simulink model "PLL_Sim_Rev1"  (R2019b)
settings: Solver=VariableStepAuto  StartTime=0.0  StopTime=10  MaxStep=100  MinStep=1e-19  RelTol=1e-2  AbsTol=1e-2
values from neighbouring files (symbols this model uses):
  C_iss = 0.1    [PLL_rev0_Plots.m]
  R = 450    [PLL_rev0_Plots.m]
  t_p = 1e-9    (= 1e-09)    [PLL_rev0_Plots.m]
  V_DD = 5    [PLL_rev0_Plots.m]
libraries: fl_lib x40, nesl_utility x21, ee_lib x15, simulink x6, simulink_extras x2, impairlib x2
settings Model: Creator=connerhannon  LastModifiedBy=connerhannon
settings SolverCC: MaxConsecutiveZCs=10000000  MaxConsecutiveMinStep=100000  ZeroCrossAlgorithm=Adaptive
settings DataIOCC: LimitDataPoints=on  MaxDataPoints=1500
settings DebuggingCC: MaxConsecutiveZCsMsg=none  MaskedZcDiagnostic=none  IgnoredZcDiagnostic=none  ArithmeticOperatorsInVariantConditions=none
settings HardwareCC: ProdBitPerLong=64  ProdHWDeviceType=Intel->x86-64 (Mac OS X)
settings ModelReferenceCC: PropagateSignalLabelsOutOfModel=off
settings SFSimCC: CustomCodeUndefinedFunction=UseInterfaceOnly
settings CodeAppCC: StateflowObjectComments=on
settings SimscapeCC: SimscapeLogType=all  SimscapeLogSimulationStatistics=on  SimscapeLogDataHistory=15000

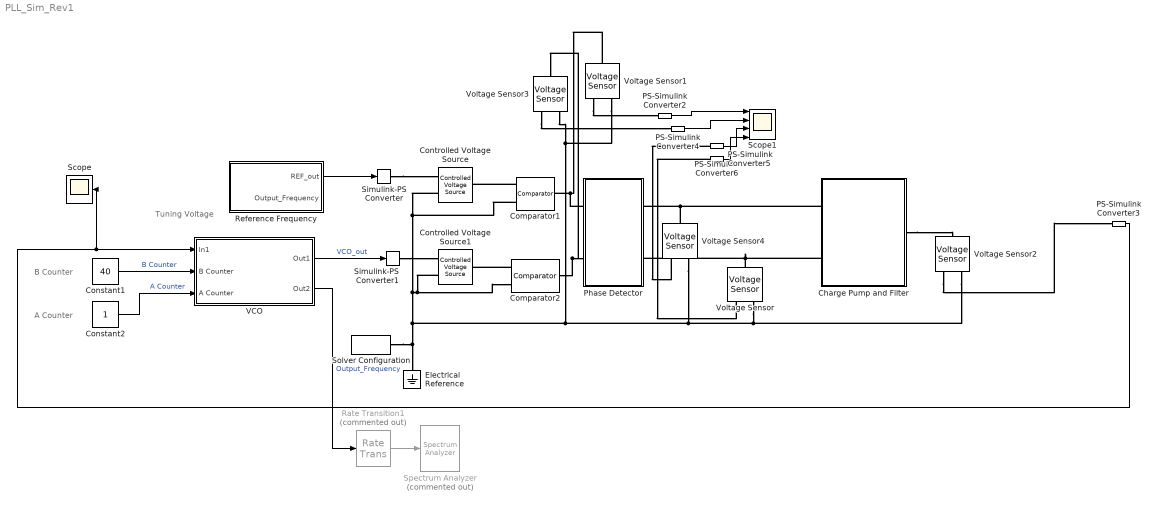
== system PLL_Sim_Rev1 ==
  note: Tuning Voltage
  note: A Counter
  note: B Counter
  Charge Pump and Filter : Subsystem  Tag=PublishSubsystem
  Comparator1 : ee_lib/Integrated Circuits/Comparator  V_OS=0 mV  V_OL=0 V  V_OH=V_DD V  C_IN=C_iss pF  R_OUT=R Ohm  Delay=t_p s
      settings: SourceProductName=Simscape Electrical  SourceProductBaseCode=PS  InternalSimscapePortConfiguration="{\"Bottom\":[],\"Left\":[{\"id\":\"p\",\"label\":\"+\",\"type\":\"foundation.electrical.electrical\"},{\"id\":\"n\",\"label\":\"-\",\"type\":\"foundation.electrical.electrical\"}],\"Right\":[{\"id\":\"J\",\"label\":\"\",\"type\":\"foundation.electrical.electrical\"}],\"Top\":[]}"
  Comparator2 : ee_lib/Integrated Circuits/Comparator  V_OS=0 mV  V_OL=0 V  V_OH=V_DD V  C_IN=C_iss pF  R_OUT=R Ohm  Delay=t_p s
      settings: SourceProductName=Simscape Electrical  SourceProductBaseCode=PS  InternalSimscapePortConfiguration="{\"Bottom\":[],\"Left\":[{\"id\":\"p\",\"label\":\"+\",\"type\":\"foundation.electrical.electrical\"},{\"id\":\"n\",\"label\":\"-\",\"type\":\"foundation.electrical.electrical\"}],\"Right\":[{\"id\":\"J\",\"label\":\"\",\"type\":\"foundation.electrical.electrical\"}],\"Top\":[]}"
  Constant1 : Constant  Value=40
  Constant2 : Constant
  Controlled Voltage Source : fl_lib/Electrical/Electrical Sources/Controlled Voltage Source
  Controlled Voltage Source1 : fl_lib/Electrical/Electrical Sources/Controlled Voltage Source
  Electrical Reference : fl_lib/Electrical/Electrical Elements/Electrical Reference
  PS-Simulink Converter{2..6} (5 alike) : nesl_utility/PS-Simulink Converter  PhysicalDomain=network_engine_domain  SubClassName=ps_output  LeftPortType=input  RightPortType=output  PseudoPeriodic=off  Frequencies=[]  Unit=inherit  AffineConversion=off
  Phase Detector : Subsystem  Tag=PublishSubsystem
  Rate Transition1 : RateTransition  Commented=on  OutPortSampleTime=1e-9
  Reference Frequency : Subsystem
  Scope : Scope
  Scope1 : Scope  NumInputPorts=4
  Simulink-PS Converter : nesl_utility/Simulink-PS Converter  PhysicalDomain=network_engine_domain  SubClassName=ps_input  LeftPortType=input  RightPortType=output  PseudoPeriodic=off  Frequencies=[]  NoiseDistribution=none  NoiseParameters=[]  Unit=1  AffineConversion=off  FilteringAndDerivatives=provide  SimscapeFilterOrder=1  InputFilterTimeConstant=0.001  UdotUserProvided=0
  Simulink-PS Converter1 : nesl_utility/Simulink-PS Converter  PhysicalDomain=network_engine_domain  SubClassName=ps_input  LeftPortType=input  RightPortType=output  PseudoPeriodic=off  Frequencies=[]  NoiseDistribution=none  NoiseParameters=[]  Unit=1  AffineConversion=off  FilteringAndDerivatives=provide  SimscapeFilterOrder=1  InputFilterTimeConstant=0.001  UdotUserProvided=0
  Solver Configuration : nesl_utility/Solver Configuration  PhysicalDomain=network_engine_domain  SubClassName=solver  LeftPortType=input  RightPortType=generic  Tones=[]  Harmonics=[]  SimulateNoise=off  Profile=off  UseLocalSampling=off  EnableSwitchedLinearOptims=on  FrequencyDomain=off  UseCCode=off  RelTol=0.001  AbsTol=1e-06  MinStep=1e-09  ToWorkspace=off  RevertToSquareIcSolve=off  NumHomotopyIterations=100  PhasorMode=off  PhasorModeNumHarmonics=1  DoDC=off  ResidualTolerance=1e-6  UseLocalSolver=off  LocalSolverChoice=NE_TRAPEZOIDAL_ADVANCER  LocalSolverSampleTime=1e-9  DoFixedCost=off  MaxNonlinIter=3  MaxModeIter=2  LinearAlgebra=auto  EquationFormulation=NE_TIME_EF  DelaysMemoryBudget=1024  AutomaticFiltering=on  FilteringTimeConstant=0.0001  PartitionStorageMethod=AS_NEEDED  PartitionMemoryBudget=1024  PartitionMethod=FAST
  Spectrum Analyzer : SpectrumAnalyzer  Commented=on
  VCO : Subsystem
  Voltage Sensor{,1..4} (5 alike) : fl_lib/Electrical/Electrical Sensors/Voltage Sensor
  wires:
  VCO/2(Out2) -> Rate Transition1/1  "Output_Frequency"
  Reference Frequency/1(REF_out) -> Simulink-PS Converter/1
  VCO/1(Out1) -> Simulink-PS Converter1/1  "VCO_out"
  Rate Transition1/1 -> Spectrum Analyzer/1
  PS-Simulink Converter2/1 -> Scope1/1
  PS-Simulink Converter4/1 -> Scope1/2
  PS-Simulink Converter6/1 -> Scope1/3
  PS-Simulink Converter5/1 -> Scope1/4
  Constant1/1 -> VCO/2(B Counter)  "B Counter"
  Constant2/1 -> VCO/3(A Counter)  "A Counter"
  PS-Simulink Converter3/1 -> Scope/1, VCO/1(In1)
  connections:
  Simulink-PS Converter1/RConn1 -- Controlled Voltage Source1/RConn1
  Simulink-PS Converter/RConn1 -- Controlled Voltage Source/RConn1
  Comparator2/LConn1 -- Controlled Voltage Source1/LConn1
  Comparator1/LConn1 -- Controlled Voltage Source/LConn1
  Phase Detector/LConn1 -- Comparator1/RConn1 -- Voltage Sensor1/LConn1
  Charge Pump and Filter/RConn1 -- Voltage Sensor2/LConn1
  Voltage Sensor2/RConn1 -- PS-Simulink Converter3/LConn1
  Charge Pump and Filter/LConn1 -- Voltage Sensor4/LConn1 -- Phase Detector/RConn1
  Charge Pump and Filter/LConn2 -- Voltage Sensor/LConn1 -- Phase Detector/RConn2
  Voltage Sensor1/RConn1 -- PS-Simulink Converter2/LConn1
  Comparator2/RConn1 -- Voltage Sensor3/LConn1 -- Phase Detector/LConn2
  Voltage Sensor3/RConn1 -- PS-Simulink Converter4/LConn1
  Voltage Sensor2/RConn2 -- Voltage Sensor/RConn2 -- Voltage Sensor4/RConn2 -- Voltage Sensor1/RConn2 -- Voltage Sensor3/RConn2 -- Comparator1/LConn2 -- Controlled Voltage Source/RConn2 -- Comparator2/LConn2 -- Controlled Voltage Source1/RConn2 -- Solver Configuration/RConn1 -- Electrical Reference/LConn1
  PS-Simulink Converter6/LConn1 -- Voltage Sensor4/RConn1
  PS-Simulink Converter5/LConn1 -- Voltage Sensor/RConn1

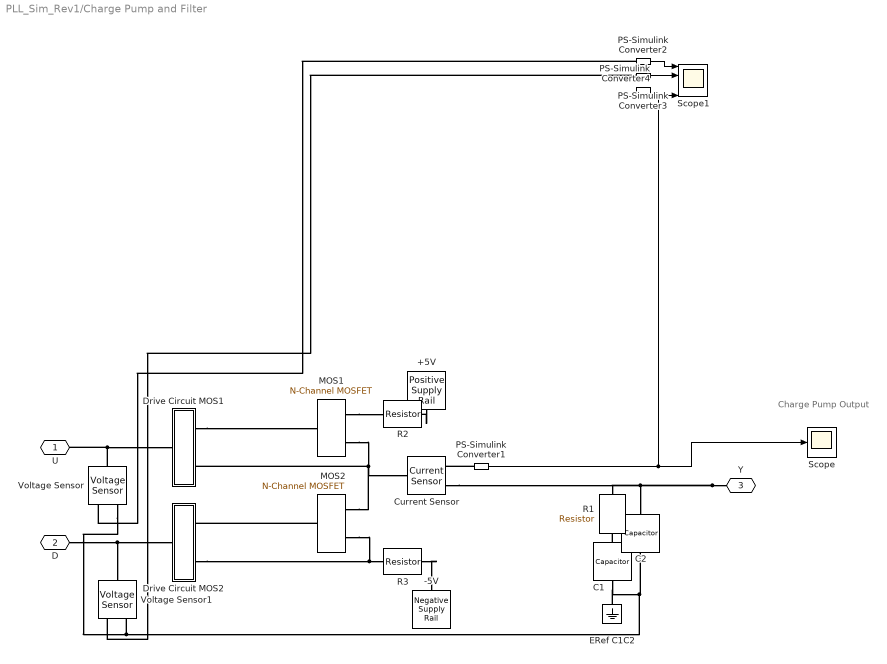
== system PLL_Sim_Rev1/Charge Pump and Filter ==
  note: Charge Pump Output
  "+5V " : ee_lib/Sources/Positive Supply Rail  v0=10 V
      settings: SourceProductName=Simscape Electrical  SourceProductBaseCode=PS  InternalSimscapePortConfiguration="{\"Bottom\":[],\"Left\":[],\"Right\":[{\"id\":\"p\",\"label\":\"\",\"type\":\"foundation.electrical.electrical\"}],\"Top\":[]}"
  -5V : ee_lib/Sources/Negative Supply Rail  v0=-10 V
      settings: SourceProductName=Simscape Electrical  SourceProductBaseCode=PS  InternalSimscapePortConfiguration="{\"Bottom\":[],\"Left\":[{\"id\":\"n\",\"label\":\"\",\"type\":\"foundation.electrical.electrical\"}],\"Right\":[],\"Top\":[]}"
  C1 : fl_lib/Electrical/Electrical Elements/Capacitor  c=82 pF  r=1e-6 Ohm  g=0 1/Ohm  i_specify=off  i_priority=High  i=0 A  i_nominal_specify=off  i_nominal_unit=A  i_nominal_value=1  v_specify=off  v_priority=High  v=0 V  v_nominal_specify=off  v_nominal_unit=V  v_nominal_value=1  vc_specify=on  vc_priority=High  vc=1 V  vc_nominal_specify=off  vc_nominal_unit=V  vc_nominal_value=1
  C2 : fl_lib/Electrical/Electrical Elements/Capacitor  c=17 pF  r=1e-6 Ohm  g=0 1/Ohm  i_specify=off  i_priority=High  i=0 A  i_nominal_specify=off  i_nominal_unit=A  i_nominal_value=1  v_specify=off  v_priority=High  v=0 V  v_nominal_specify=off  v_nominal_unit=V  v_nominal_value=1  vc_specify=on  vc_priority=High  vc=1 V  vc_nominal_specify=off  vc_nominal_unit=V  vc_nominal_value=1
  Current Sensor : fl_lib/Electrical/Electrical Sensors/Current Sensor
  Drive Circuit MOS1 : Subsystem
  Drive Circuit MOS2 : Subsystem
  ERef C1C2 : fl_lib/Electrical/Electrical Elements/Electrical Reference
  MOS1 : ee_lib/Semiconductors & Converters/N-Channel MOSFET  parameterization=1  prmDatasheet=1  prmEquCoeff=1  Beta=5 A/V^2  Rds=1000 Ohm  Id=2.5e-4 A  Vgs=5 V  Vth=1 V  lam=0 1/V  Tmeas=25 degC  RS=1 Ohm  RD=1 Ohm  C_param=1  C_GS=270 pF  C_GD=80 pF  C_DS=0 pF  C_iss=0.35 pF  C_rss=0.1 pF  C_oss=0 pF  C_GS_vec=[ 270 300 290 280 295 255 ] pF  C_GD_vec=[ 450 400 300 190 95 55 ] pF  C_DS_vec=[ 450 410 390 230 175 115 ] pF  C_iss_vec=[ 720 700 590 470 390 310 ] pF  C_rss_vec=[ 450 400 300 190 95 55 ] pF  C_oss_vec=[ 900 810 690 420 270 170 ] pF  C_Vds_vec=[ 0.1 0.3 1 3 10 30 ] V  V_GS_for_cap_data=NaN V  charge_linearity_param=1  C_OX=200 pF  V_C_OX=-0.5 V  IsDiode=0 A  Vbi=0.6 V  n=1  Cj0Diode=0 pF  TT=50e-9 s  dVth_dT=-6 mV/K  Rds_T2=0.037 Ohm  Tmeas2=125 degC  BEXDatasheet=-1.5  BEXEquCoeff=-1.5  etaisDatasheet=3  etaisEquCoeff=3  TdeviceDatasheet=25 degC  TdeviceEquCoeff=25 degC  thermal_network_parameterization=ee.enum.thermalNetworkTopology.cauer  Rth=[0, 10] K/W  Rth_Foster=[4, 6] K/W  thermal_mass_parameterization=ee.enum.thermalNetwork.timeconstant  thermal_mass=[0, 1] J/K  thermal_mass_Foster=[1.5, 3] J/K  thermal_time_constant=[0, 10] s  thermal_time_constant_Foster=[6, 18] s  thermal_mass_initial_temperatures=[25, 25] degC  betaref=18 A/V^2  Vfbref=-1.1 V  gamma=3.5 V^0.50000  phib2ref=1 V  thesatref=0.4 1/V  alpha=0  Vp=5e-2 V  thesrref=0 1/V  m=8  Tref=25 degC  Cox=1500 pF  Cgso=100 pF  Cgdo=14 pF  Rsref=2e-3 Ohm  Rdref=0.17 Ohm  Rgref=8.4 Ohm  Isref=5.2e-13 A  Cj0=480 pF  Tprm=1  etabet=1.3  Stvfb=5e-4 V/K  Stphib=-8.5e-4 V/K  etasat=1.04  etasr=0.65  etar=0.95  etais=3  Tsim=25 degC  T0=[25, 25] degC
      settings: SourceProductName=Simscape Electrical
  MOS2 : ee_lib/Semiconductors & Converters/N-Channel MOSFET  parameterization=1  prmDatasheet=1  prmEquCoeff=1  Beta=5 A/V^2  Rds=1000 Ohm  Id=2.5e-4 A  Vgs=5 V  Vth=1 V  lam=0 1/V  Tmeas=25 degC  RS=1 Ohm  RD=1 Ohm  C_param=1  C_GS=270 pF  C_GD=80 pF  C_DS=0 pF  C_iss=0.35 pF  C_rss=0.1 pF  C_oss=0 pF  C_GS_vec=[ 270 300 290 280 295 255 ] pF  C_GD_vec=[ 450 400 300 190 95 55 ] pF  C_DS_vec=[ 450 410 390 230 175 115 ] pF  C_iss_vec=[ 720 700 590 470 390 310 ] pF  C_rss_vec=[ 450 400 300 190 95 55 ] pF  C_oss_vec=[ 900 810 690 420 270 170 ] pF  C_Vds_vec=[ 0.1 0.3 1 3 10 30 ] V  V_GS_for_cap_data=NaN V  charge_linearity_param=1  C_OX=200 pF  V_C_OX=-0.5 V  IsDiode=0 A  Vbi=0.6 V  n=1  Cj0Diode=0 pF  TT=50e-9 s  dVth_dT=-6 mV/K  Rds_T2=0.037 Ohm  Tmeas2=125 degC  BEXDatasheet=-1.5  BEXEquCoeff=-1.5  etaisDatasheet=3  etaisEquCoeff=3  TdeviceDatasheet=25 degC  TdeviceEquCoeff=25 degC  thermal_network_parameterization=ee.enum.thermalNetworkTopology.cauer  Rth=[0, 10] K/W  Rth_Foster=[4, 6] K/W  thermal_mass_parameterization=ee.enum.thermalNetwork.timeconstant  thermal_mass=[0, 1] J/K  thermal_mass_Foster=[1.5, 3] J/K  thermal_time_constant=[0, 10] s  thermal_time_constant_Foster=[6, 18] s  thermal_mass_initial_temperatures=[25, 25] degC  betaref=18 A/V^2  Vfbref=-1.1 V  gamma=3.5 V^0.50000  phib2ref=1 V  thesatref=0.4 1/V  alpha=0  Vp=5e-2 V  thesrref=0 1/V  m=8  Tref=25 degC  Cox=1500 pF  Cgso=100 pF  Cgdo=14 pF  Rsref=2e-3 Ohm  Rdref=0.17 Ohm  Rgref=8.4 Ohm  Isref=5.2e-13 A  Cj0=480 pF  Tprm=1  etabet=1.3  Stvfb=5e-4 V/K  Stphib=-8.5e-4 V/K  etasat=1.04  etasr=0.65  etar=0.95  etais=3  Tsim=25 degC  T0=[25, 25] degC
      settings: SourceProductName=Simscape Electrical
  PS-Simulink Converter{1..4} (4 alike) : nesl_utility/PS-Simulink Converter  PhysicalDomain=network_engine_domain  SubClassName=ps_output  LeftPortType=input  RightPortType=output  PseudoPeriodic=off  Frequencies=[]  Unit=inherit  AffineConversion=off
  R1 : ee_lib/Passive/Resistor  R=23 kOhm  R_tol=5  enable_R_tol=0  tol_distribution=1  nSigma=4  enable_operating_limits=0  operating_limit_action=2  max_working_voltage=100 V  power_rating=1 W  enable_faults=0  fault_action=1  R_faulted=Inf Ohm  enable_temporal_fault=0  t_fault=1 s  enable_behavioral_fault=0  max_permissible_current=1 A  t_fail_on_current=1 s  noise_mode=0  sample_time=0.001 s  repeatability=1  auto_seed=66516699  user_seed=0  Tdevice=25 degC  alpha=3.93e-3 1/K  Tmeas=25 degC  thermal_mass=100 J/K  power_derating_T1=70 degC  power_derating_T2=155 degC  operating_temperature_range_vec=[-50, 150] degC  temperature_specify=off  temperature_priority=High  temperature=298.15 K  temperature_nominal_specify=off  temperature_nominal_unit=K  temperature_nominal_value=1
      settings: SourceProductName=Simscape Electrical
  R2 : ee_lib/Passive/Resistor  R=40 kOhm  R_tol=5  enable_R_tol=0  tol_distribution=1  nSigma=4  enable_operating_limits=0  operating_limit_action=2  max_working_voltage=100 V  power_rating=1 W  enable_faults=0  fault_action=1  R_faulted=Inf Ohm  enable_temporal_fault=0  t_fault=1 s  enable_behavioral_fault=0  max_permissible_current=1 A  t_fail_on_current=1 s  noise_mode=0  sample_time=0.001 s  repeatability=1  auto_seed=4226521513  user_seed=0  Tdevice=25 degC  alpha=3.93e-3 1/K  Tmeas=25 degC  thermal_mass=100 J/K  power_derating_T1=70 degC  power_derating_T2=155 degC  operating_temperature_range_vec=[-50, 150] degC  temperature_specify=off  temperature_priority=High  temperature=298.15 K  temperature_nominal_specify=off  temperature_nominal_unit=K  temperature_nominal_value=1
      settings: SourceProductName=Simscape Electrical
  R3 : ee_lib/Passive/Resistor  R=40 kOhm  R_tol=5  enable_R_tol=0  tol_distribution=1  nSigma=4  enable_operating_limits=0  operating_limit_action=2  max_working_voltage=100 V  power_rating=1 W  enable_faults=0  fault_action=1  R_faulted=Inf Ohm  enable_temporal_fault=0  t_fault=1 s  enable_behavioral_fault=0  max_permissible_current=1 A  t_fail_on_current=1 s  noise_mode=0  sample_time=0.001 s  repeatability=1  auto_seed=717982854  user_seed=0  Tdevice=25 degC  alpha=3.93e-3 1/K  Tmeas=25 degC  thermal_mass=100 J/K  power_derating_T1=70 degC  power_derating_T2=155 degC  operating_temperature_range_vec=[-50, 150] degC  temperature_specify=off  temperature_priority=High  temperature=298.15 K  temperature_nominal_specify=off  temperature_nominal_unit=K  temperature_nominal_value=1
      settings: SourceProductName=Simscape Electrical
  Scope : Scope
  Scope1 : Scope  NumInputPorts=4
  Voltage Sensor : fl_lib/Electrical/Electrical Sensors/Voltage Sensor
  Voltage Sensor1 : fl_lib/Electrical/Electrical Sensors/Voltage Sensor
  U : PMIOPort  Side=Left
  D : PMIOPort  Port=2  Side=Left
  Y : PMIOPort  Port=3  Side=Right
  wires:
  PS-Simulink Converter1/1 -> Scope1/4, Scope/1
  PS-Simulink Converter2/1 -> Scope1/1
  PS-Simulink Converter3/1 -> Scope1/2
  connections:
  C1/LConn1 -- R1/RConn1
  MOS2/RConn2 -- Drive Circuit MOS2/RConn2 -- R3/LConn1
  "+5V "/RConn1 -- R2/LConn1
  MOS1/RConn1 -- R2/RConn1
  R3/RConn1 -- -5V/LConn1
  MOS1/RConn2 -- MOS2/RConn1 -- Current Sensor/LConn1 -- Drive Circuit MOS1/RConn2
  PS-Simulink Converter1/LConn1 -- Current Sensor/RConn1
  Voltage Sensor/RConn2 -- C2/RConn1 -- C1/RConn1 -- ERef C1C2/LConn1 -- Voltage Sensor1/RConn2
  MOS2/LConn1 -- Drive Circuit MOS2/RConn1
  Drive Circuit MOS1/RConn1 -- MOS1/LConn1
  PS-Simulink Converter2/LConn1 -- Voltage Sensor/RConn1
  PS-Simulink Converter3/LConn1 -- Voltage Sensor1/RConn1
  Voltage Sensor/LConn1 -- Drive Circuit MOS1/LConn1 -- U/RConn1
  D/RConn1 -- Voltage Sensor1/LConn1 -- Drive Circuit MOS2/LConn1
  Y/RConn1 -- Current Sensor/RConn2 -- R1/LConn1 -- C2/LConn1

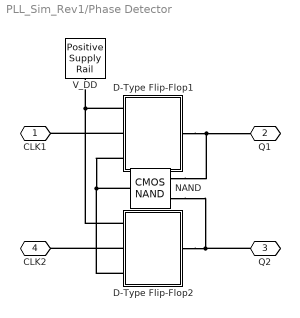
== system PLL_Sim_Rev1/Phase Detector ==
  D-Type Flip-Flop1 : Subsystem  mask(D-Type Flip-Flop){C_iss=C_iss, t_p=t_p, V_DD=V_DD, R=R}
      mask prompts: C_iss "Gate input capacitance (pF)"; t_p "Gate propagation delay (s)"; V_DD "Supply voltage (V)"; R "Gate effective output resistance (ohms)"
      mask help: Behavioral model of a D-type flip-flop built from Simscape(TM) Electrical(TM) library components.
  D-Type Flip-Flop2 : Subsystem  mask(D-Type Flip-Flop){C_iss=C_iss, t_p=t_p, V_DD=V_DD, R=R}
      mask prompts: C_iss "Gate input capacitance (pF)"; t_p "Gate propagation delay (s)"; V_DD "Supply voltage (V)"; R "Gate effective output resistance (ohms)"
      mask help: Behavioral model of a D-type flip-flop built from Simscape(TM) Electrical(TM) library components.
  NAND : ee_lib/Integrated Circuits/Logic/CMOS NAND  V_IL=0.4*V_DD V  V_IH=0.6*V_DD V  C_IN=C_iss pF  output_type=1  V_OL=0 V  V_OH=V_DD V  V_CC=5 V  V_meas=5 V  R_OUT=R Ohm  R_OH=[ 25 250 ] Ohm  I_OH=63 mA  R_OL=[ 30 800 ] Ohm  I_OL=-45 mA  Delay=t_p s  Ron=5 Ohm  Vf=0.6 V  output_state=1
      settings: SourceProductName=Simscape Electrical  SourceProductBaseCode=PS  InternalSimscapePortConfiguration="{\"Bottom\":[],\"Left\":[{\"id\":\"A\",\"label\":\"\",\"type\":\"foundation.electrical.electrical\"},{\"id\":\"B\",\"label\":\"\",\"type\":\"foundation.electrical.electrical\"}],\"Right\":[{\"id\":\"J\",\"label\":\"\",\"type\":\"foundation.electrical.electrical\"}],\"Top\":[]}"
  V_DD : ee_lib/Sources/Positive Supply Rail  v0=V_DD V
      settings: SourceProductName=Simscape Electrical  SourceProductBaseCode=PS  InternalSimscapePortConfiguration="{\"Bottom\":[],\"Left\":[],\"Right\":[{\"id\":\"p\",\"label\":\"\",\"type\":\"foundation.electrical.electrical\"}],\"Top\":[]}"
  CLK1 : PMIOPort  Side=Left
  Q1 : PMIOPort  Port=2  Side=Right
  Q2 : PMIOPort  Port=3  Side=Right
  CLK2 : PMIOPort  Port=4  Side=Left
  connections:
  D-Type Flip-Flop1/LConn1 -- D-Type Flip-Flop2/LConn1 -- V_DD/RConn1
  D-Type Flip-Flop1/LConn3 -- D-Type Flip-Flop2/LConn3 -- NAND/RConn1
  NAND/LConn2 -- D-Type Flip-Flop1/RConn1 -- Q1/RConn1
  NAND/LConn1 -- D-Type Flip-Flop2/RConn1 -- Q2/RConn1
  D-Type Flip-Flop2/LConn2 -- CLK2/RConn1
  D-Type Flip-Flop1/LConn2 -- CLK1/RConn1

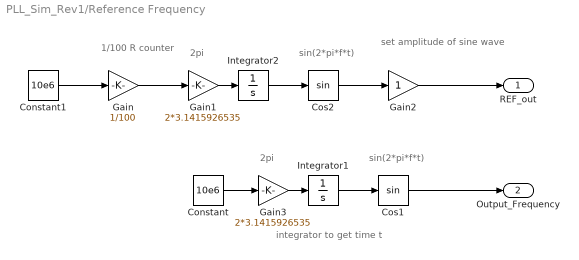
== system PLL_Sim_Rev1/Reference Frequency ==
  note: set amplitude of sine wave
  note: 1/100
      | R counter
  note: integrator to get time t
  note: sin(2*pi*f*t)
  note: 2pi
  note: sin(2*pi*f*t)
  note: 2pi
  Constant : Constant  Value=10e6
  Constant1 : Constant  Value=10e6
  Cos1 : Trigonometry  OutputSignalType=real
  Cos2 : Trigonometry  OutputSignalType=real
  Gain : Gain  Gain=1/100
  Gain1 : Gain  Gain=2*3.1415926535
  Gain2 : Gain
  Gain3 : Gain  Gain=2*3.1415926535
  Integrator1 : Integrator
  Integrator2 : Integrator
  REF_out : Outport
  "Output_Frequency " : Outport  Port=2
  wires:
  Cos1/1 -> "Output_Frequency "/1
  Gain3/1 -> Integrator1/1
  Integrator1/1 -> Cos1/1
  Constant/1 -> Gain3/1
  Constant1/1 -> Gain/1
  Gain1/1 -> Integrator2/1
  Integrator2/1 -> Cos2/1
  Gain/1 -> Gain1/1
  Cos2/1 -> Gain2/1
  Gain2/1 -> REF_out/1

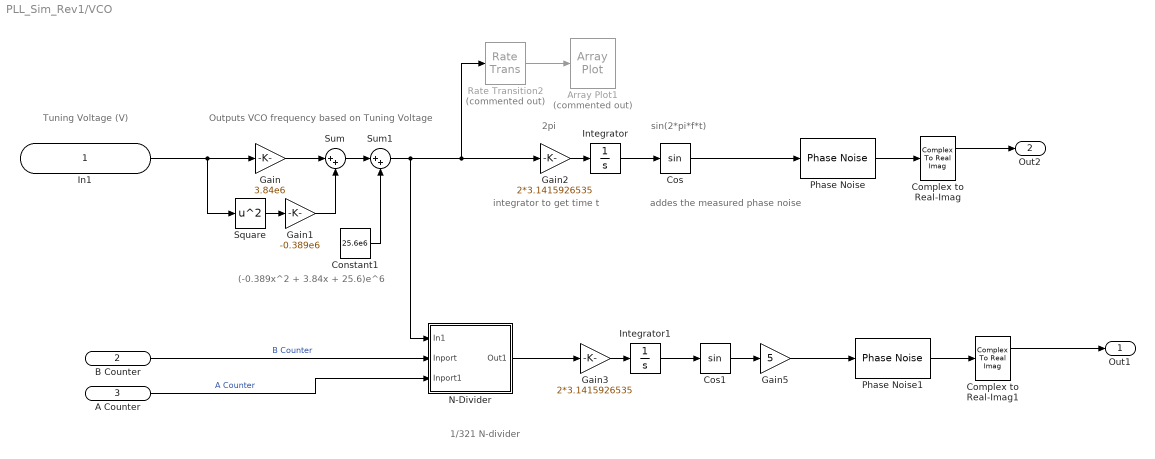
== system PLL_Sim_Rev1/VCO ==
  note: 1/321
      | N-divider
  note: Tuning Voltage
      | (V)
  note: 2pi
  note: sin(2*pi*f*t)
  note: integrator to get time t
  note: (-0.389x^2 + 3.84x + 25.6)e^6
  note: addes the measured phase noise
  note: Outputs VCO frequency based on Tuning Voltage
  In1 : Inport
  B Counter : Inport  Port=2
  A Counter : Inport  Port=3
  Array Plot1 : ArrayPlot  Commented=on
  Complex to Real-Imag : ComplexToRealImag
  Complex to Real-Imag1 : ComplexToRealImag
  Constant1 : Constant  Value=25.6e6
  Cos : Trigonometry  OutputSignalType=complex
  Cos1 : Trigonometry  OutputSignalType=complex
  Gain : Gain  Gain=3.84e6
  Gain1 : Gain  Gain=-0.389e6
  Gain2 : Gain  Gain=2*3.1415926535
  Gain3 : Gain  Gain=2*3.1415926535
  Gain5 : Gain  Gain=5
  Integrator : Integrator
  Integrator1 : Integrator
  N-Divider : Subsystem
  Phase Noise : impairlib/Phase Noise  Level=[ -36, -73, -83, -90, -112 ]  FrequencyOffset=[ 100, 400, 1000, 5000, 250000]  SampleRate=550000  RandomStream=mt19937ar with seed  Seed=1e6  SimulateUsing=Interpreted execution
      settings: SourceProductName=SerDes Toolbox  SourceProductBaseCode=SX
  Phase Noise1 : impairlib/Phase Noise  Level=[ -36, -73, -83, -90, -112 ]  FrequencyOffset=[ 100, 400, 1000, 5000, 250000]  SampleRate=550000  RandomStream=mt19937ar with seed  Seed=1e6  SimulateUsing=Interpreted execution
      settings: SourceProductName=SerDes Toolbox  SourceProductBaseCode=SX
  Rate Transition2 : RateTransition  Commented=on  OutPortSampleTime=1/1000000000
  Square : Math  Operator=square  SignedPower=off  SaturateOnIntegerOverflow=on
  Sum : Sum  Inputs=|++
  Sum1 : Sum  Inputs=|++
  Out1 : Outport
  Out2 : Outport  Port=2
  wires:
  Gain1/1 -> Sum/2
  Gain/1 -> Sum/1
  Square/1 -> Gain1/1
  Integrator/1 -> Cos/1
  Constant1/1 -> Sum1/2
  Phase Noise/1 -> Complex to Real-Imag/1
  Sum/1 -> Sum1/1
  Cos/1 -> Phase Noise/1
  In1/1 -> Square/1, Gain/1
  Gain2/1 -> Integrator/1
  Gain3/1 -> Integrator1/1
  Phase Noise1/1 -> Complex to Real-Imag1/1
  Cos1/1 -> Gain5/1
  Integrator1/1 -> Cos1/1
  Complex to Real-Imag1/1 -> Out1/1
  Complex to Real-Imag/1 -> Out2/1
  Gain5/1 -> Phase Noise1/1
  Sum1/1 -> N-Divider/1(In1), Rate Transition2/1, Gain2/1
  B Counter/1 -> N-Divider/2(Inport)  "B Counter"
  A Counter/1 -> N-Divider/3(Inport1)  "A Counter"
  N-Divider/1(Out1) -> Gain3/1
  Rate Transition2/1 -> Array Plot1/1

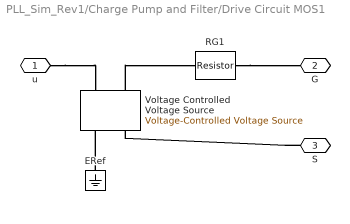
== system PLL_Sim_Rev1/Charge Pump and Filter/Drive Circuit MOS1 ==
  ERef : fl_lib/Electrical/Electrical Elements/Electrical Reference
  RG1 : ee_lib/Passive/Resistor  R=40 kOhm  R_tol=5  enable_R_tol=0  tol_distribution=1  nSigma=4  enable_operating_limits=0  operating_limit_action=2  max_working_voltage=100 V  power_rating=1 W  enable_faults=0  fault_action=1  R_faulted=Inf Ohm  enable_temporal_fault=0  t_fault=1 s  enable_behavioral_fault=0  max_permissible_current=1 A  t_fail_on_current=1 s  noise_mode=0  sample_time=0.001 s  repeatability=1  auto_seed=1254062075  user_seed=0  Tdevice=25 degC  alpha=3.93e-3 1/K  Tmeas=25 degC  thermal_mass=100 J/K  power_derating_T1=70 degC  power_derating_T2=155 degC  operating_temperature_range_vec=[-50, 150] degC  temperature_specify=off  temperature_priority=High  temperature=298.15 K  temperature_nominal_specify=off  temperature_nominal_unit=K  temperature_nominal_value=1
      settings: SourceProductName=Simscape Electrical
  Voltage Controlled Voltage Source : fl_lib/Electrical/Electrical Sources/Voltage-Controlled Voltage Source  K=1  v1_specify=off  v1_priority=High  v1=0 V  v1_nominal_specify=off  v1_nominal_unit=V  v1_nominal_value=1  v2_specify=off  v2_priority=High  v2=0 V  v2_nominal_specify=off  v2_nominal_unit=V  v2_nominal_value=1
      settings: SourceProductName=Simscape  SourceProductBaseCode=SS  InternalSimscapePortConfiguration="{\"Bottom\":[],\"Left\":[{\"id\":\"p1\",\"label\":\"+\",\"type\":\"foundation.electrical.electrical\"},{\"id\":\"p2\",\"label\":\"+\",\"type\":\"foundation.electrical.electrical\"}],\"Right\":[{\"id\":\"n1\",\"label\":\"-\",\"type\":\"foundation.electrical.electrical\"},{\"id\":\"n2\",\"label\":\"-\",\"type\":\"foundation.electrical.electrical\"}],\"Top\":[]}"
  u : PMIOPort  Side=Left
  G : PMIOPort  Port=2  Side=Right
  S : PMIOPort  Port=3  Side=Right
  connections:
  u/RConn1 -- Voltage Controlled Voltage Source/LConn1
  S/RConn1 -- Voltage Controlled Voltage Source/RConn2
  RG1/RConn1 -- G/RConn1
  Voltage Controlled Voltage Source/LConn2 -- RG1/LConn1
  ERef/LConn1 -- Voltage Controlled Voltage Source/RConn1

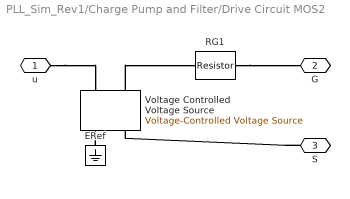
== system PLL_Sim_Rev1/Charge Pump and Filter/Drive Circuit MOS2 ==
  ERef : fl_lib/Electrical/Electrical Elements/Electrical Reference
  RG1 : ee_lib/Passive/Resistor  R=40 kOhm  R_tol=5  enable_R_tol=0  tol_distribution=1  nSigma=4  enable_operating_limits=0  operating_limit_action=2  max_working_voltage=100 V  power_rating=1 W  enable_faults=0  fault_action=1  R_faulted=Inf Ohm  enable_temporal_fault=0  t_fault=1 s  enable_behavioral_fault=0  max_permissible_current=1 A  t_fail_on_current=1 s  noise_mode=0  sample_time=0.001 s  repeatability=1  auto_seed=1853927660  user_seed=0  Tdevice=25 degC  alpha=3.93e-3 1/K  Tmeas=25 degC  thermal_mass=100 J/K  power_derating_T1=70 degC  power_derating_T2=155 degC  operating_temperature_range_vec=[-50, 150] degC  temperature_specify=off  temperature_priority=High  temperature=298.15 K  temperature_nominal_specify=off  temperature_nominal_unit=K  temperature_nominal_value=1
      settings: SourceProductName=Simscape Electrical
  Voltage Controlled Voltage Source : fl_lib/Electrical/Electrical Sources/Voltage-Controlled Voltage Source  K=1  v1_specify=off  v1_priority=High  v1=0 V  v1_nominal_specify=off  v1_nominal_unit=V  v1_nominal_value=1  v2_specify=off  v2_priority=High  v2=0 V  v2_nominal_specify=off  v2_nominal_unit=V  v2_nominal_value=1
      settings: SourceProductName=Simscape  SourceProductBaseCode=SS  InternalSimscapePortConfiguration="{\"Bottom\":[],\"Left\":[{\"id\":\"p1\",\"label\":\"+\",\"type\":\"foundation.electrical.electrical\"},{\"id\":\"p2\",\"label\":\"+\",\"type\":\"foundation.electrical.electrical\"}],\"Right\":[{\"id\":\"n1\",\"label\":\"-\",\"type\":\"foundation.electrical.electrical\"},{\"id\":\"n2\",\"label\":\"-\",\"type\":\"foundation.electrical.electrical\"}],\"Top\":[]}"
  u : PMIOPort  Side=Left
  G : PMIOPort  Port=2  Side=Right
  S : PMIOPort  Port=3  Side=Right
  connections:
  ERef/LConn1 -- Voltage Controlled Voltage Source/RConn1
  Voltage Controlled Voltage Source/LConn2 -- RG1/LConn1
  RG1/RConn1 -- G/RConn1
  S/RConn1 -- Voltage Controlled Voltage Source/RConn2
  u/RConn1 -- Voltage Controlled Voltage Source/LConn1

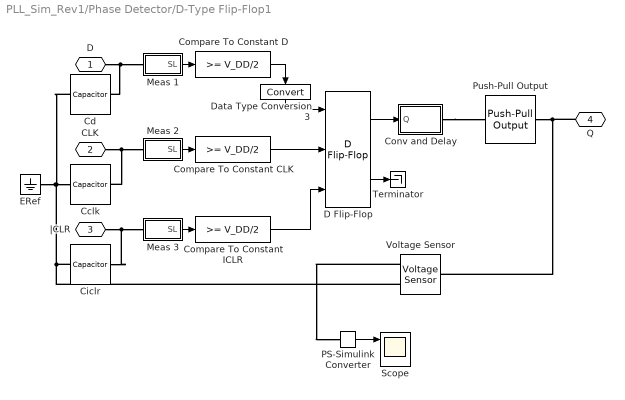
== system PLL_Sim_Rev1/Phase Detector/D-Type Flip-Flop1 ==
  Cclk : fl_lib/Electrical/Electrical Elements/Capacitor  c=C_iss pF  r=1e-06 Ohm  g=0 1/Ohm  i_specify=off  i_priority=High  i=0 A  i_nominal_specify=off  i_nominal_unit=A  i_nominal_value=1  v_specify=off  v_priority=High  v=0 V  v_nominal_specify=off  v_nominal_unit=V  v_nominal_value=1  vc_specify=on  vc_priority=High  vc=0 V  vc_nominal_specify=off  vc_nominal_unit=V  vc_nominal_value=1
  Cd : fl_lib/Electrical/Electrical Elements/Capacitor  c=C_iss pF  r=1e-06 Ohm  g=0 1/Ohm  i_specify=off  i_priority=High  i=0 A  i_nominal_specify=off  i_nominal_unit=A  i_nominal_value=1  v_specify=off  v_priority=High  v=0 V  v_nominal_specify=off  v_nominal_unit=V  v_nominal_value=1  vc_specify=on  vc_priority=High  vc=0 V  vc_nominal_specify=off  vc_nominal_unit=V  vc_nominal_value=1
  Ciclr : fl_lib/Electrical/Electrical Elements/Capacitor  c=C_iss pF  r=1e-06 Ohm  g=0 1/Ohm  i_specify=off  i_priority=High  i=0 A  i_nominal_specify=off  i_nominal_unit=A  i_nominal_value=1  v_specify=off  v_priority=High  v=0 V  v_nominal_specify=off  v_nominal_unit=V  v_nominal_value=1  vc_specify=on  vc_priority=High  vc=0 V  vc_nominal_specify=off  vc_nominal_unit=V  vc_nominal_value=1
  Compare To Constant CLK : simulink/Logic and Bit Operations/Compare To Constant  relop=>=  const=V_DD/2  OutDataTypeStr=boolean
  Compare To Constant D : simulink/Logic and Bit Operations/Compare To Constant  relop=>=  const=V_DD/2  OutDataTypeStr=boolean
  Compare To Constant ICLR : simulink/Logic and Bit Operations/Compare To Constant  relop=>=  const=V_DD/2  OutDataTypeStr=boolean
  Conv and Delay : Subsystem
  D Flip-Flop : simulink_extras/Flip Flops/D Flip-Flop
      settings: SourceProductName=Simulink
  Data Type Conversion3 : DataTypeConversion
  ERef : fl_lib/Electrical/Electrical Elements/Electrical Reference
  Meas 1 : Subsystem
  Meas 2 : Subsystem
  Meas 3 : Subsystem
  PS-Simulink Converter : nesl_utility/PS-Simulink Converter  PhysicalDomain=network_engine_domain  SubClassName=ps_output  LeftPortType=input  RightPortType=output  PseudoPeriodic=off  Frequencies=[]  Unit=inherit  AffineConversion=off
  Push-Pull Output : ee_lib/Integrated Circuits/Push-Pull Output  k=-V_DD V  c=-1  output_type=1  V_neg=0 V  V_pos=V_DD V  V_meas=[ 0 5 ] V  R_OUT=R Ohm  R_OH=[ 25 250 ] Ohm  I_OH=63 mA  R_OL=[ 30 800 ] Ohm  I_OL=-45 mA  Delay=0 s  Ron=5 Ohm  Vf=0.6 V  V0=0 V  X0=0
      settings: SourceProductName=Simscape Electrical  SourceProductBaseCode=PS  InternalSimscapePortConfiguration="{\"Bottom\":[],\"Left\":[{\"id\":\"X\",\"label\":\"X\",\"type\":\"input\"}],\"Right\":[{\"id\":\"J\",\"label\":\"\",\"type\":\"foundation.electrical.electrical\"}],\"Top\":[]}"
  Scope : Scope  NumInputPorts=3
  Terminator : Terminator
  Voltage Sensor : fl_lib/Electrical/Electrical Sensors/Voltage Sensor
  D : PMIOPort  Side=Left
  CLK : PMIOPort  Port=2  Side=Left
  |CLR : PMIOPort  Port=3  Side=Left
  Q : PMIOPort  Port=4  Side=Right
  wires:
  Data Type Conversion3/1 -> D Flip-Flop/1
  Compare To Constant ICLR/1 -> D Flip-Flop/3
  Compare To Constant CLK/1 -> D Flip-Flop/2
  D Flip-Flop/2 -> Terminator/1
  Compare To Constant D/1 -> Data Type Conversion3/1
  Meas 3/1(SL) -> Compare To Constant ICLR/1
  Meas 2/1(SL) -> Compare To Constant CLK/1
  Meas 1/1(SL) -> Compare To Constant D/1
  D Flip-Flop/1 -> Conv and Delay/1(Q)
  PS-Simulink Converter/1 -> Scope/1
  connections:
  |CLR/RConn1 -- Ciclr/LConn1 -- Meas 3/LConn1
  Voltage Sensor/LConn1 -- Q/RConn1 -- Push-Pull Output/RConn1
  CLK/RConn1 -- Meas 2/LConn1 -- Cclk/LConn1
  D/RConn1 -- Cd/LConn1 -- Meas 1/LConn1
  ERef/LConn1 -- Voltage Sensor/RConn2 -- Ciclr/RConn1 -- Cd/RConn1 -- Cclk/RConn1
  Conv and Delay/RConn1 -- Push-Pull Output/LConn1
  Voltage Sensor/RConn1 -- PS-Simulink Converter/LConn1

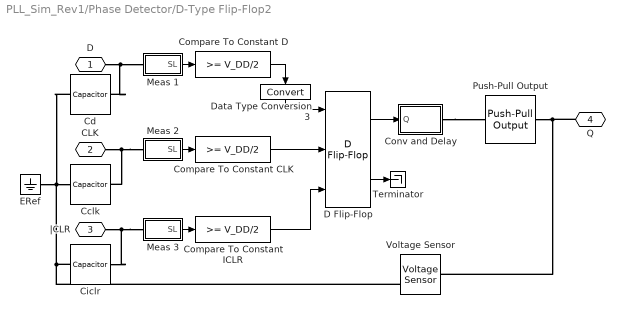
== system PLL_Sim_Rev1/Phase Detector/D-Type Flip-Flop2 ==
  Cclk : fl_lib/Electrical/Electrical Elements/Capacitor  c=C_iss pF  r=1e-06 Ohm  g=0 1/Ohm  i_specify=off  i_priority=High  i=0 A  i_nominal_specify=off  i_nominal_unit=A  i_nominal_value=1  v_specify=off  v_priority=High  v=0 V  v_nominal_specify=off  v_nominal_unit=V  v_nominal_value=1  vc_specify=on  vc_priority=High  vc=0 V  vc_nominal_specify=off  vc_nominal_unit=V  vc_nominal_value=1
  Cd : fl_lib/Electrical/Electrical Elements/Capacitor  c=C_iss pF  r=1e-06 Ohm  g=0 1/Ohm  i_specify=off  i_priority=High  i=0 A  i_nominal_specify=off  i_nominal_unit=A  i_nominal_value=1  v_specify=off  v_priority=High  v=0 V  v_nominal_specify=off  v_nominal_unit=V  v_nominal_value=1  vc_specify=on  vc_priority=High  vc=0 V  vc_nominal_specify=off  vc_nominal_unit=V  vc_nominal_value=1
  Ciclr : fl_lib/Electrical/Electrical Elements/Capacitor  c=C_iss pF  r=1e-06 Ohm  g=0 1/Ohm  i_specify=off  i_priority=High  i=0 A  i_nominal_specify=off  i_nominal_unit=A  i_nominal_value=1  v_specify=off  v_priority=High  v=0 V  v_nominal_specify=off  v_nominal_unit=V  v_nominal_value=1  vc_specify=on  vc_priority=High  vc=0 V  vc_nominal_specify=off  vc_nominal_unit=V  vc_nominal_value=1
  Compare To Constant CLK : simulink/Logic and Bit Operations/Compare To Constant  relop=>=  const=V_DD/2  OutDataTypeStr=boolean
  Compare To Constant D : simulink/Logic and Bit Operations/Compare To Constant  relop=>=  const=V_DD/2  OutDataTypeStr=boolean
  Compare To Constant ICLR : simulink/Logic and Bit Operations/Compare To Constant  relop=>=  const=V_DD/2  OutDataTypeStr=boolean
  Conv and Delay : Subsystem
  D Flip-Flop : simulink_extras/Flip Flops/D Flip-Flop
      settings: SourceProductName=Simulink
  Data Type Conversion3 : DataTypeConversion
  ERef : fl_lib/Electrical/Electrical Elements/Electrical Reference
  Meas 1 : Subsystem
  Meas 2 : Subsystem
  Meas 3 : Subsystem
  Push-Pull Output : ee_lib/Integrated Circuits/Push-Pull Output  k=-V_DD V  c=-1  output_type=1  V_neg=0 V  V_pos=V_DD V  V_meas=[ 0 5 ] V  R_OUT=R Ohm  R_OH=[ 25 250 ] Ohm  I_OH=63 mA  R_OL=[ 30 800 ] Ohm  I_OL=-45 mA  Delay=0 s  Ron=5 Ohm  Vf=0.6 V  V0=0 V  X0=0
      settings: SourceProductName=Simscape Electrical  SourceProductBaseCode=PS  InternalSimscapePortConfiguration="{\"Bottom\":[],\"Left\":[{\"id\":\"X\",\"label\":\"X\",\"type\":\"input\"}],\"Right\":[{\"id\":\"J\",\"label\":\"\",\"type\":\"foundation.electrical.electrical\"}],\"Top\":[]}"
  Terminator : Terminator
  Voltage Sensor : fl_lib/Electrical/Electrical Sensors/Voltage Sensor
  D : PMIOPort  Side=Left
  CLK : PMIOPort  Port=2  Side=Left
  |CLR : PMIOPort  Port=3  Side=Left
  Q : PMIOPort  Port=4  Side=Right
  wires:
  D Flip-Flop/1 -> Conv and Delay/1(Q)
  Meas 1/1(SL) -> Compare To Constant D/1
  Meas 2/1(SL) -> Compare To Constant CLK/1
  Meas 3/1(SL) -> Compare To Constant ICLR/1
  Compare To Constant D/1 -> Data Type Conversion3/1
  D Flip-Flop/2 -> Terminator/1
  Compare To Constant CLK/1 -> D Flip-Flop/2
  Compare To Constant ICLR/1 -> D Flip-Flop/3
  Data Type Conversion3/1 -> D Flip-Flop/1
  connections:
  Conv and Delay/RConn1 -- Push-Pull Output/LConn1
  Ciclr/RConn1 -- Voltage Sensor/RConn2 -- Cclk/RConn1 -- ERef/LConn1 -- Cd/RConn1
  Cd/LConn1 -- Meas 1/LConn1 -- D/RConn1
  Meas 2/LConn1 -- Cclk/LConn1 -- CLK/RConn1
  Push-Pull Output/RConn1 -- Q/RConn1 -- Voltage Sensor/LConn1
  Meas 3/LConn1 -- |CLR/RConn1 -- Ciclr/LConn1

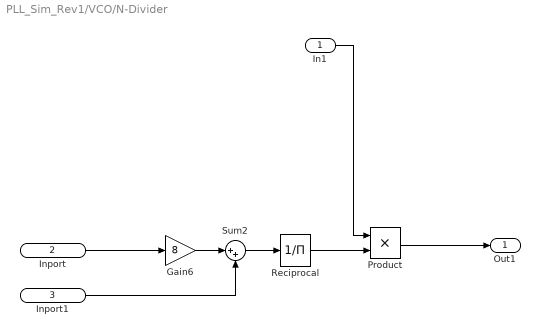
== system PLL_Sim_Rev1/VCO/N-Divider ==
  In1 : Inport
  Inport : Inport  Port=2
  Inport1 : Inport  Port=3
  Gain6 : Gain  Gain=8
  Product : Product
  Reciprocal : Product  Inputs=/
  Sum2 : Sum  Inputs=|++
  Out1 : Outport
  wires:
  Product/1 -> Out1/1
  Inport/1 -> Gain6/1
  Sum2/1 -> Reciprocal/1
  Gain6/1 -> Sum2/1
  Reciprocal/1 -> Product/2
  In1/1 -> Product/1
  Inport1/1 -> Sum2/2

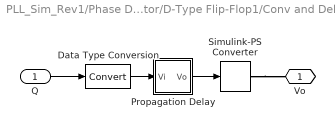
== system PLL_Sim_Rev1/Phase Detector/D-Type Flip-Flop1/Conv and Delay ==
  Q : Inport
  Data Type Conversion : DataTypeConversion
  Propagation Delay : Subsystem
  Simulink-PS Converter : nesl_utility/Simulink-PS Converter  PhysicalDomain=network_engine_domain  SubClassName=ps_input  LeftPortType=input  RightPortType=output  PseudoPeriodic=off  Frequencies=[]  NoiseDistribution=none  NoiseParameters=[]  Unit=V  AffineConversion=off  FilteringAndDerivatives=zero  SimscapeFilterOrder=1  InputFilterTimeConstant=.001  UdotUserProvided=0
  Vo : PMIOPort  Side=Right
  wires:
  Propagation Delay/1(Vo) -> Simulink-PS Converter/1
  Data Type Conversion/1 -> Propagation Delay/1(Vi)
  Q/1 -> Data Type Conversion/1
  connections:
  Simulink-PS Converter/RConn1 -- Vo/RConn1

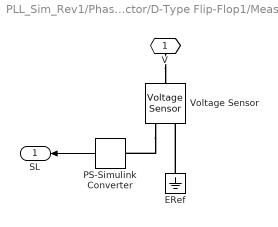
== system PLL_Sim_Rev1/Phase Detector/D-Type Flip-Flop1/Meas 1 ==
  ERef : fl_lib/Electrical/Electrical Elements/Electrical Reference
  PS-Simulink Converter : nesl_utility/PS-Simulink Converter  PhysicalDomain=network_engine_domain  SubClassName=ps_output  LeftPortType=input  RightPortType=output  PseudoPeriodic=off  Frequencies=[]  Unit=V  AffineConversion=off
  Voltage Sensor : fl_lib/Electrical/Electrical Sensors/Voltage Sensor
  V : PMIOPort  Side=Left
  SL : Outport  VectorParamsAs1DForOutWhenUnconnected=off
  wires:
  PS-Simulink Converter/1 -> SL/1
  connections:
  Voltage Sensor/RConn1 -- PS-Simulink Converter/LConn1
  ERef/LConn1 -- Voltage Sensor/RConn2
  V/RConn1 -- Voltage Sensor/LConn1

== system PLL_Sim_Rev1/Phase Detector/D-Type Flip-Flop1/Meas 2 ==
  ERef : fl_lib/Electrical/Electrical Elements/Electrical Reference
  PS-Simulink Converter : nesl_utility/PS-Simulink Converter  PhysicalDomain=network_engine_domain  SubClassName=ps_output  LeftPortType=input  RightPortType=output  PseudoPeriodic=off  Frequencies=[]  Unit=V  AffineConversion=off
  Voltage Sensor : fl_lib/Electrical/Electrical Sensors/Voltage Sensor
  V : PMIOPort  Side=Left
  SL : Outport  VectorParamsAs1DForOutWhenUnconnected=off
  wires:
  PS-Simulink Converter/1 -> SL/1
  connections:
  V/RConn1 -- Voltage Sensor/LConn1
  ERef/LConn1 -- Voltage Sensor/RConn2
  Voltage Sensor/RConn1 -- PS-Simulink Converter/LConn1

== system PLL_Sim_Rev1/Phase Detector/D-Type Flip-Flop1/Meas 3 ==
  ERef : fl_lib/Electrical/Electrical Elements/Electrical Reference
  PS-Simulink Converter : nesl_utility/PS-Simulink Converter  PhysicalDomain=network_engine_domain  SubClassName=ps_output  LeftPortType=input  RightPortType=output  PseudoPeriodic=off  Frequencies=[]  Unit=V  AffineConversion=off
  Voltage Sensor : fl_lib/Electrical/Electrical Sensors/Voltage Sensor
  V : PMIOPort  Side=Left
  SL : Outport  VectorParamsAs1DForOutWhenUnconnected=off
  wires:
  PS-Simulink Converter/1 -> SL/1
  connections:
  Voltage Sensor/RConn1 -- PS-Simulink Converter/LConn1
  ERef/LConn1 -- Voltage Sensor/RConn2
  V/RConn1 -- Voltage Sensor/LConn1

== system PLL_Sim_Rev1/Phase Detector/D-Type Flip-Flop2/Conv and Delay ==
  Q : Inport
  Data Type Conversion : DataTypeConversion
  Propagation Delay : Subsystem
  Simulink-PS Converter : nesl_utility/Simulink-PS Converter  PhysicalDomain=network_engine_domain  SubClassName=ps_input  LeftPortType=input  RightPortType=output  PseudoPeriodic=off  Frequencies=[]  NoiseDistribution=none  NoiseParameters=[]  Unit=V  AffineConversion=off  FilteringAndDerivatives=zero  SimscapeFilterOrder=1  InputFilterTimeConstant=.001  UdotUserProvided=0
  Vo : PMIOPort  Side=Right
  wires:
  Q/1 -> Data Type Conversion/1
  Data Type Conversion/1 -> Propagation Delay/1(Vi)
  Propagation Delay/1(Vo) -> Simulink-PS Converter/1
  connections:
  Simulink-PS Converter/RConn1 -- Vo/RConn1

== system PLL_Sim_Rev1/Phase Detector/D-Type Flip-Flop2/Meas 1 ==
  ERef : fl_lib/Electrical/Electrical Elements/Electrical Reference
  PS-Simulink Converter : nesl_utility/PS-Simulink Converter  PhysicalDomain=network_engine_domain  SubClassName=ps_output  LeftPortType=input  RightPortType=output  PseudoPeriodic=off  Frequencies=[]  Unit=V  AffineConversion=off
  Voltage Sensor : fl_lib/Electrical/Electrical Sensors/Voltage Sensor
  V : PMIOPort  Side=Left
  SL : Outport  VectorParamsAs1DForOutWhenUnconnected=off
  wires:
  PS-Simulink Converter/1 -> SL/1
  connections:
  V/RConn1 -- Voltage Sensor/LConn1
  ERef/LConn1 -- Voltage Sensor/RConn2
  Voltage Sensor/RConn1 -- PS-Simulink Converter/LConn1

== system PLL_Sim_Rev1/Phase Detector/D-Type Flip-Flop2/Meas 2 ==
  ERef : fl_lib/Electrical/Electrical Elements/Electrical Reference
  PS-Simulink Converter : nesl_utility/PS-Simulink Converter  PhysicalDomain=network_engine_domain  SubClassName=ps_output  LeftPortType=input  RightPortType=output  PseudoPeriodic=off  Frequencies=[]  Unit=V  AffineConversion=off
  Voltage Sensor : fl_lib/Electrical/Electrical Sensors/Voltage Sensor
  V : PMIOPort  Side=Left
  SL : Outport  VectorParamsAs1DForOutWhenUnconnected=off
  wires:
  PS-Simulink Converter/1 -> SL/1
  connections:
  Voltage Sensor/RConn1 -- PS-Simulink Converter/LConn1
  ERef/LConn1 -- Voltage Sensor/RConn2
  V/RConn1 -- Voltage Sensor/LConn1

== system PLL_Sim_Rev1/Phase Detector/D-Type Flip-Flop2/Meas 3 ==
  ERef : fl_lib/Electrical/Electrical Elements/Electrical Reference
  PS-Simulink Converter : nesl_utility/PS-Simulink Converter  PhysicalDomain=network_engine_domain  SubClassName=ps_output  LeftPortType=input  RightPortType=output  PseudoPeriodic=off  Frequencies=[]  Unit=V  AffineConversion=off
  Voltage Sensor : fl_lib/Electrical/Electrical Sensors/Voltage Sensor
  V : PMIOPort  Side=Left
  SL : Outport  VectorParamsAs1DForOutWhenUnconnected=off
  wires:
  PS-Simulink Converter/1 -> SL/1
  connections:
  V/RConn1 -- Voltage Sensor/LConn1
  ERef/LConn1 -- Voltage Sensor/RConn2
  Voltage Sensor/RConn1 -- PS-Simulink Converter/LConn1

== system PLL_Sim_Rev1/Phase Detector/D-Type Flip-Flop1/Conv and Delay/Propagation Delay ==
  Vi : Inport
  1/propagation delay : Gain  Gain=1/t_p
  Integrator : Integrator
  Sum : Sum  Inputs=|+-
  Vo : Outport  VectorParamsAs1DForOutWhenUnconnected=off
  wires:
  1/propagation delay/1 -> Integrator/1
  Sum/1 -> 1/propagation delay/1
  Vi/1 -> Sum/1
  Integrator/1 -> Sum/2, Vo/1

== system PLL_Sim_Rev1/Phase Detector/D-Type Flip-Flop2/Conv and Delay/Propagation Delay ==
  Vi : Inport
  1/propagation delay : Gain  Gain=1/t_p
  Integrator : Integrator
  Sum : Sum  Inputs=|+-
  Vo : Outport  VectorParamsAs1DForOutWhenUnconnected=off
  wires:
  Integrator/1 -> Vo/1, Sum/2
  Vi/1 -> Sum/1
  Sum/1 -> 1/propagation delay/1
  1/propagation delay/1 -> Integrator/1
